simulink model "satelit"  (R2017b)
settings: Solver=ode4  StartTime=0.0  StopTime=723000  FixedStep=2  RelTol=1e-3
settings Model: Creator=squirrel  LastModifiedBy=squirrel

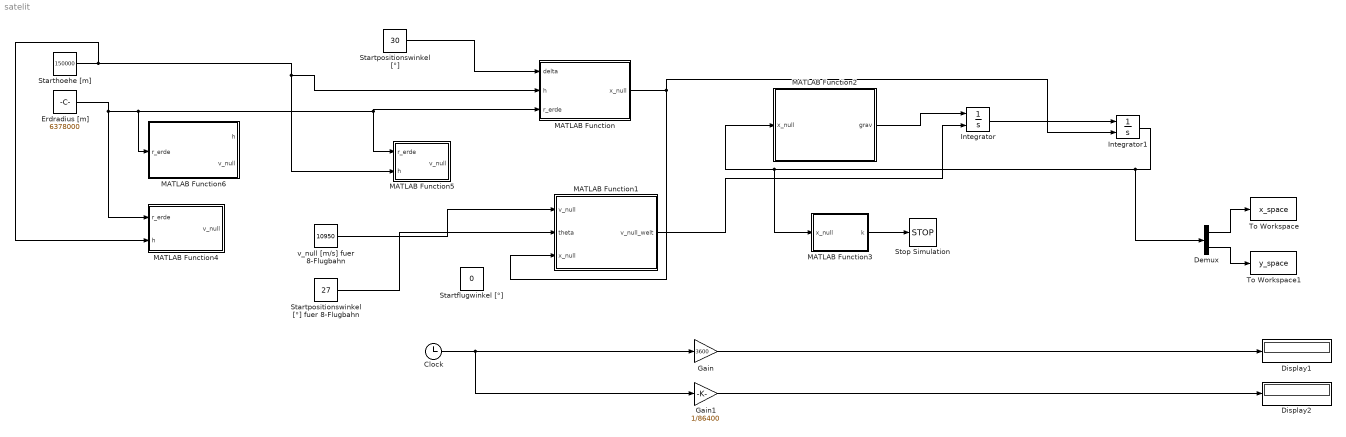
== system satelit ==
  Clock : Clock
  Demux : Demux  Outputs=2
  Display1 : Display
  Display2 : Display
  Erdradius [m] : Constant  Value=6378000
  Gain : Gain  Gain=3600
  Gain1 : Gain  Gain=1/86400
  Integrator : Integrator  InitialConditionSource=external
  Integrator1 : Integrator  InitialConditionSource=external
  MATLAB Function : MATLAB Function  TreatAsAtomicUnit=on
  MATLAB Function1 : MATLAB Function  TreatAsAtomicUnit=on
  MATLAB Function2 : MATLAB Function  TreatAsAtomicUnit=on
  MATLAB Function3 : MATLAB Function  TreatAsAtomicUnit=on
  MATLAB Function4 : MATLAB Function  TreatAsAtomicUnit=on
  MATLAB Function5 : MATLAB Function  TreatAsAtomicUnit=on
  MATLAB Function6 : MATLAB Function  TreatAsAtomicUnit=on
  Startflugwinkel [°] : Constant  Value=0
  Starthoehe [m] : Constant  Value=150000
  Startpositionswinkel [°] : Constant  Value=30
  Startpositionswinkel [°] fuer 8-Flugbahn : Constant  Value=27
  Stop Simulation : Stop
  To Workspace : ToWorkspace  VariableName=x_space  SampleTime=-1
  To Workspace1 : ToWorkspace  VariableName=y_space  SampleTime=-1
  v_null [m/s] fuer 8-Flugbahn : Constant  Value=10950
  wires:
  Clock/1 -> Gain1/1, Gain/1
  Gain/1 -> Display1/1
  Demux/1 -> To Workspace/1
  Demux/2 -> To Workspace1/1
  MATLAB Function2/1(grav) -> Integrator/1
  MATLAB Function1/1(v_null_welt) -> Integrator/2
  Integrator/1 -> Integrator1/1
  MATLAB Function/1(x_null) -> MATLAB Function1/3(x_null), Integrator1/2
  Integrator1/1 -> Demux/1, MATLAB Function3/1(x_null), MATLAB Function2/1(x_null)
  MATLAB Function3/1(k) -> Stop Simulation/1
  Startpositionswinkel [°]/1 -> MATLAB Function/1(delta)
  Starthoehe [m]/1 -> MATLAB Function4/2(h), MATLAB Function/2(h), MATLAB Function5/2(h)
  Gain1/1 -> Display2/1
  Erdradius [m]/1 -> MATLAB Function4/1(r_erde), MATLAB Function6/1(r_erde), MATLAB Function/3(r_erde), MATLAB Function5/1(r_erde)
  v_null [m/s] fuer 8-Flugbahn/1 -> MATLAB Function1/1(v_null)
  Startpositionswinkel [°] fuer 8-Flugbahn/1 -> MATLAB Function1/2(theta)

== matlab function satelit/MATLAB Function1 ==
  data: v_null input; v_null_welt output; theta input; x_null input
function v_null_welt = vStart(v_null, theta, x_null)
% Funktion zur Berechnung der Startgeschwindigkeit v_null
n = x_null / norm(x_null); % Einheitsvektor in Normalenrichtung
t = [n(2); -n(1)]; % Einheitsvektor in Tangentialrichtung

theta_bogen = (theta / 180) * pi;  % Startflugwinkel [Radien]

vn = sin(theta_bogen) * n; % Normalkomponente der Startgeschwindigkeit
vt = cos(theta_bogen) * t; % Tangentialkomponente der Startgeschwindigkeit

v_null_welt = (vt + vn) * v_null; % v_null_welt [m/s]

== matlab function satelit/MATLAB Function ==
  data: delta input; x_null output; h input; r_erde input
function x_null = startposition(delta, h, r_erde)
% Funktion zur Berechnung des Startpositionsvektors x_null
delta_bogen = (delta / 180) * pi; % Startpositionswinkel [Radien]
hyp = h + r_erde; % Distanz vom Satellit zum Erdmittelpunkt [m]
x_null = [hyp * cos(delta_bogen); hyp * sin(delta_bogen)]; % Startpositionsvektor (Spaltenvektor)

== matlab function satelit/MATLAB Function2 ==
  data: x_null input; grav output
function grav = Gravitation(x_null)
% Funktion zur Berechnung der Gravitation
G = 66.743 * 10^-12; % Gravitationskonstante [m³/(kg * s²)]
m_e = 5.9736 * 10^24; % Erdmasse [kg]
m_m = 7.3480 * 10^22; % Mondmasse [kg]
x_mond = [0; -380000000]; % Monposition [m]
e_se = x_null / norm(x_null); % Einheitsvektor des Satelliten
e_mond = (x_mond - x_null) / norm(x_mond - x_null); % Einheitsvektor zwischen Satellit und Mond
r = norm(x_null); % Abstand von Erdmittelpunkt zum Satellit [m]
r_sat_mond = norm(x_mond - x_null); % Abstand von Satellit zum Mond [m]

grav_erde = -(G * (m_e / (r^2)) * e_se); % negative Gravitationskraft zwischen Erde und Satellit
grav_mond = G * (m_m / (r_sat_mond^2) * e_mond); % Gravitationskraft zwischen Satellit und Mond
grav = grav_erde + grav_mond; % Summe beider Gravitationen ergibt die Gesamtgravitation auf Satellit

== matlab function satelit/MATLAB Function3 ==
  data: x_null input; k output
function k = Kontakt(x_null)
r_erde = 6378000; % Erdradius [m]
l = norm(x_null); % Entfernung des Satelliten zum Erdmittelpunkt [m]
if(l <= r_erde)
    k = 1;
else
    k = 0;
end

== matlab function satelit/MATLAB Function4 ==
  data: r_erde input; v_null output; h input
function v_null = kreisbahn(r_erde, h)
% Funktion zur Berechnung von 1a) Kreisbahn in gleicher Hoehe
G = 66.743 * 10^-12;  % Gravitationskonstante [m³/(kg * s²)]
m_e = 5.9736 * 10^24; % Erdmasse [kg]
v_null = sqrt(G * m_e / (h + r_erde)); % Startgeschwindigkeit [m/s] fuer Kreisbahn in gleicher Hoehe

== matlab function satelit/MATLAB Function5 ==
  data: r_erde input; v_null output; h input
function v_null = flucht(r_erde, h)
% Funktion zur Berechnung von 1b) Satellit entflieht gerade der Erde
% dauerhaft
G = 66.743 * 10^-12; % Gravitationskonstante [m³/(kg * s²)]
m_e = 5.9736 * 10^24; % Erdmasse [kg]
v_null = sqrt(2 * G * m_e / (h + r_erde)); % Startgeschwindigkeit [m/s], um Erde gerade dauerhaft zu entfliehen

== matlab function satelit/MATLAB Function6 ==
  data: h output; v_null output; r_erde input
function [h, v_null] = geobahn(r_erde)
% Funktion zur Berechnung von 1c) Kreisbahn dauert genau 1 Tag
t = 86400; % Zeit := 1 Tag [s]
G = 66.743 * 10^-12; % Gravitationskonstante [m³/(kg * s²)]
m_e = 5.9736 * 10^24; % Erdmasse [kg]

h = nthroot((G * m_e * (t/(2 * pi))^2), 3) - r_erde; % Starthoehe des Sateliten, so dass eine Kreisbahn genau 1 Tag dauert
v_null = (2 * pi * (h + r_erde)) / t; % Geschwingikeit, so dass eine Kreisbahn genau 1 Tag dauert
